simulink model "Closeloop"  (R2024b)
settings: Solver=FixedStepAuto  StartTime=0.0  StopTime=10.0  RelTol=1e-3  EnableMultiTasking=on
libraries: legoev3lib x4
settings Model: ExtModeTrigDuration=2  Creator=franc  LastModifiedBy=franc
settings SolverCC: PositivePriorityOrder=on
settings OptimizationCC: DefaultParameterBehavior=Inlined  EnhancedBackFolding=on  PassReuseOutputArgsAs=Individual arguments  ZeroExternalMemoryAtStartup=off  ZeroInternalMemoryAtStartup=off  MaxStackSize=64  OptimizeBlockOrder=speed  DifferentSizesBufferReuse=on  OptimizationCustomize=off  EfficientTunableParamExpr=on
settings DebuggingCC: ParameterTunabilityLossMsg=error
settings HardwareCC: ProdBitPerPointer=32  ProdBitPerSizeT=32  ProdBitPerPtrDiffT=32  ProdLargestAtomicInteger=Long  ProdWordSize=32  ProdHWDeviceType=ARM Compatible->ARM 9  UseEmbeddedCoderFeatures=off  UseSimulinkCoderFeatures=off
settings SFSimCC: MATLABDynamicMemAlloc=off
settings RTWCC: Description=Embedded Coder  SystemTargetFile=ert.tlc  HardwareBoard=LEGO MINDSTORMS EV3  TLCOptions="-aInlineSetEventsForThisBaseRateFcn=TLC_FALSE -aSuppressMultiTaskScheduler=TLC_FALSE  -aRateBasedStepFcn=0"  TemplateMakefile=ert_default_tmf  Toolchain=Sourcery G++ Lite v2009q3
settings CodeAppCC: ForceParamTrailComments=on  IgnoreCustomStorageClasses=off  OperatorAnnotations=on  SimulinkDataObjDesc=on  SFDataObjDesc=on  InsertBlockDesc=on
settings ERTTargetCC: SupportContinuousTime=on  SupportNonInlinedSFcns=on  SupportVariableSizeSignals=on  ExtModeTransport=2  ExtModeStaticAlloc=on  ExtModeMexFile=ext_xcp  ExtModeIntrfLevel=Level2 - Open

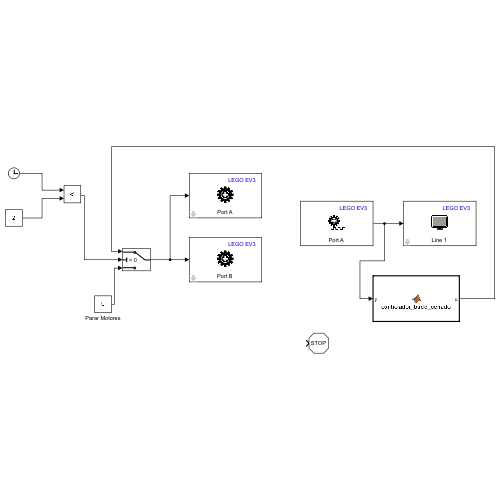
[thumbnail: Simulink's stored preview of the top-level diagram]
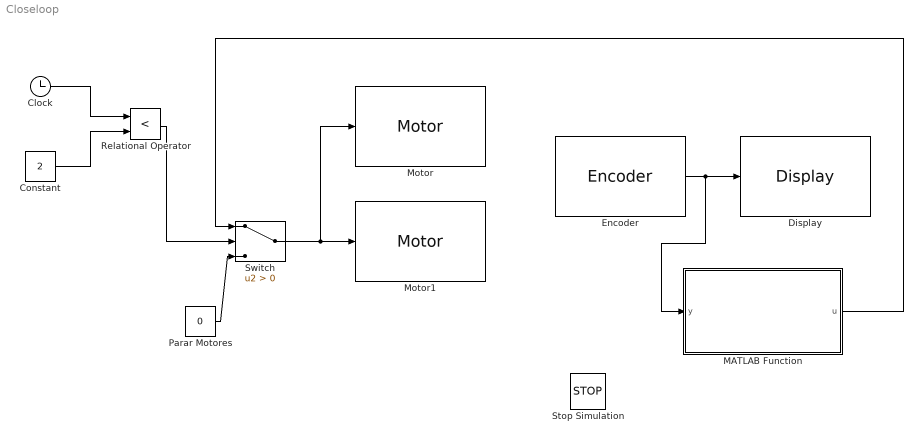
== system Closeloop ==
  Clock : Clock
  Constant : Constant  Value=2
  Display : legoev3lib/Display  slcdLine=1  slcdFormat=Decimal
  Encoder : legoev3lib/Encoder  portNumber=A  opMode=Reset at each sample time  sampleTime=0.1
  MATLAB Function : MATLAB Function  TreatAsAtomicUnit=on
  Motor : legoev3lib/Motor  sportNumber=A  sstopAction=Brake
  Motor1 : legoev3lib/Motor  sportNumber=B  sstopAction=Brake
  Parar Motores : Constant  Value=0
  Relational Operator : RelationalOperator  Operator=<  OutDataTypeStr=boolean  RndMeth=Simplest  InputSameDT=off
  Stop Simulation : Stop
  Switch : Switch  Criteria=u2 > Threshold  SaturateOnIntegerOverflow=off  InputSameDT=off
  wires:
  Clock/1 -> Relational Operator/1
  Constant/1 -> Relational Operator/2
  Encoder/1 -> Display/1, MATLAB Function/1(y)
  Relational Operator/1 -> Switch/2
  Parar Motores/1 -> Switch/3
  Switch/1 -> Motor1/1, Motor/1
  MATLAB Function/1(u) -> Switch/1

== matlab function Closeloop/MATLAB Function ==
  data: y input; u output
function u = controlador_bucle_cerrado(y)
    persistent iteraciones;
    persistent energia_motor;
    
    salida_deseada = 860; % Referencia
    max_potencia = 100;   % Límite superior de la potencia
    min_potencia = -100;  % Límite inferior de la potencia
    
    % Inicialización de variables persistentes como double
    if isempty(iteraciones)
        iteraciones = double(0);
    end
    if isempty(energia_motor)
        energia_motor = double(50); % Valor inicial de la energía del motor
    end
    
    % Asegurar que y es de tipo double
    y = double(y);
    
    % Cálculo del error
    error = salida_deseada - y;
    
    % Aplicación del control con conversión a double
    if iteraciones == 0
        u = double(energia_motor); % Primera iteración usa el valor inicial
    else
        u = double(max(min_potencia, min(max_potencia, error))); % Saturar la señal de control
    end
    
    % Convertir iteraciones a double antes de la suma
    iteraciones = double(iteraciones + 1);
    
    % Detener motor después de 2000 iteraciones
    if iteraciones >= 2000
        u = double(0);
    end
end
